simulink model "test"  (R2024a)
settings: Solver=VariableStepAuto  StartTime=0.0  StopTime=10.0  RelTol=1e-3
settings Model: Creator=thistle  LastModifiedBy=thistle

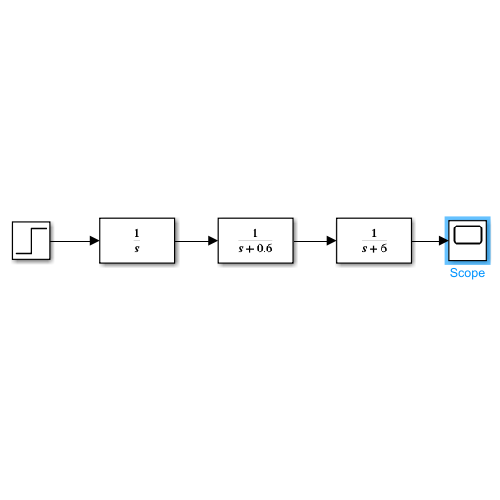
[thumbnail: Simulink's stored preview of the top-level diagram]
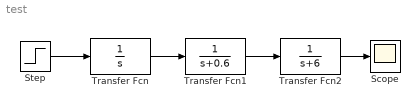
== system test ==
  Scope : Scope
  Step : Step  SampleTime=0
  Transfer Fcn : TransferFcn  Denominator=[1 0]
  Transfer Fcn1 : TransferFcn  Denominator=[1 0.6]
  Transfer Fcn2 : TransferFcn  Denominator=[1 6]
  wires:
  Step/1 -> Transfer Fcn/1
  Transfer Fcn/1 -> Transfer Fcn1/1
  Transfer Fcn1/1 -> Transfer Fcn2/1
  Transfer Fcn2/1 -> Scope/1
